simulink model "untitl3ed"  (R2021a)
settings: Solver=VariableStepAuto  StartTime=0.0  StopTime=10  RelTol=1e-3
undefined symbols (not defined in the file or in its folder): DiscIntNeverNeededParam, Ion, Lithium, sigbuilder_block
libraries: spsCurrentMeasurementLib x3, spsControlledCurrentSourceLib x2, spspowerguiLib x1, spsBatteryLib x1, spsControlledVoltageSourceLib x1, spsDiodeLib x1, spsFuelCellStackLib x1, spsSeriesRLCBranchLib x1, pid_lib x1
settings Model: Creator=leonardopalacios  LastModifiedBy=leonardopalacios
settings SolverCC: ZeroCrossAlgorithm=Adaptive
settings DebuggingCC: IgnoredZcDiagnostic=none

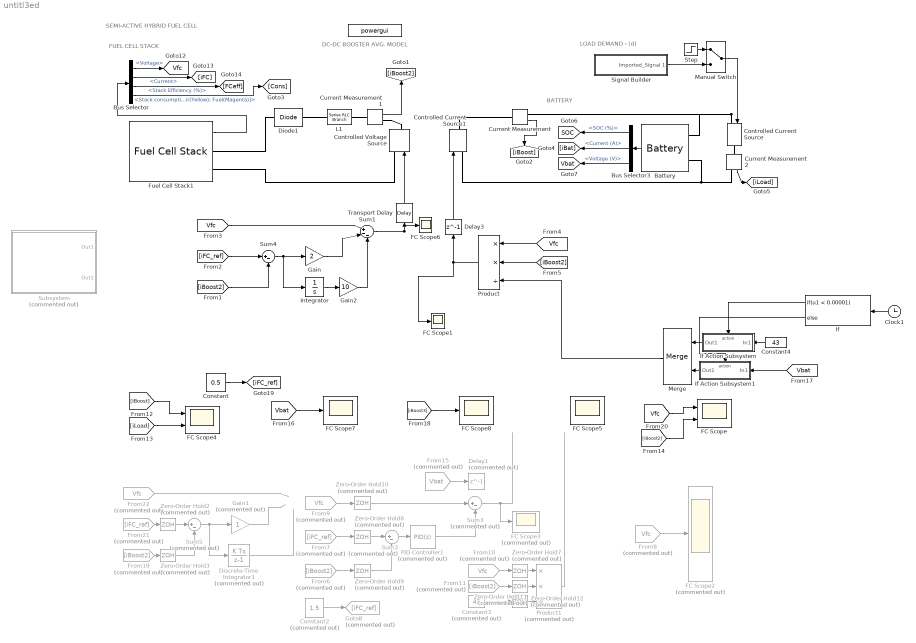
== system untitl3ed ==
  note: FUEL CELL STACK
  note: DC-DC BOOSTER AVG. MODEL
  note: BATTERY
  note: SEMI-ACTIVE HYBRID FUEL CELL
  note: LOAD DEMAND - (d)
  " " : spspowerguiLib/powergui  Priority=1  SimulationMode=Continuous  SampleTime=50e-6  frequency=60  Iterations=50  frequencyindice=0  Pbase=100e6  ErrMax=1e-4  UnitsV=kV  UnitsW=MW  buscounter=0  FunctionMessages=off  echomessages=off  EnableUseOfTLC=off  CurrentSourceSwitches=off  DisableSnubberDevices=off  DisableRonSwitches=off  DisableVfSwitches=off  DisplayEquations=off  AutomaticDiscreteSolvers=off  SolverType=Tustin/Backward Euler (TBE)  Interpol=off  ExternalGateDelay=off  methode=off  Ts=10  x0status=blocks  SPID=off  SwTol=0  HookPort=off  NonlinearTolerance=1e-4  nMaxIteration=100  ContinueOnMaxIteration=off  RestoreLinks=warning  ResistiveCurrentMeasurement=off  Frange=[0:2:500]  Ylog=off  Xlog=on  ShowGrid=off  save=off  variable=ZData  structure=0  ZoomFFT=off  StartTime=0.0  cycles=1  DisplayStyle=1  fundamental=60  FreqAxis=off  MaxFrequency=1000  frequencyindicesteady=1  RmsSteady=1  display=off
  Battery : spsBatteryLib/Battery  BatType=Lithium-Ion  ShowTempParam=off  ThermalPreset=no  ShowAgeParam=off  NomV=40  NomQ=2.2  SOC=50  Batt_Tr=30  PresetModel=on  MaxQ=2.2  MinV=30  FullV=46.5595  Dis_rate=0.95652  R=0.18182  Normal_OP=1.9896  expZone="[43.2154     0.108087]"  current=[6.5 13 32.5]  Units=Time  Tci=20  NomT=25  T2=0  MaxQ2=2.208  FullV2=3.45  Normal_OP2=2.8  expZone2="[3.22        0.23]"  Rca=0.6  ti=1000  Dp=0  Neq0=0  Tsim=1e6  Ta1=25  Qeol=5.4*0.9  Reol=0.013333*1.2  Char_age=[2.3478, 3]  Dis_age=[2.3478, 10]  N1=1500  N2=10500  N3=1000  N4=1400  Ta2=45  N5=950
  Bus Selector : BusSelector  OutputSignals=Voltage,Current,Stack Efficiency (%),Stack consumption (Standard lpm) [Air(Yellow); Fuel(Magenta)]
  Bus Selector3 : BusSelector  OutputSignals=SOC (%),Current (A),Voltage (V)
  Clock1 : Clock
  Constant : Constant  Value=0.5
  Constant2 : Constant  Commented=on  Value=1.5
  Constant3 : Constant  Commented=on  Value=43
  Constant4 : Constant  Value=43
  Controlled Current Source : spsControlledCurrentSourceLib/Controlled Current Source  Initialize=off  Source_Type=DC  Amplitude=0  Phase=0  Frequency=0  Measurements=Current
  Controlled Current Source1 : spsControlledCurrentSourceLib/Controlled Current Source  Initialize=on  Source_Type=DC  Amplitude=0  Phase=0  Frequency=0  Measurements=Current
  Controlled Voltage Source : spsControlledVoltageSourceLib/Controlled Voltage Source  Initialize=on  Source_Type=DC  Amplitude=32.5  Phase=0  Frequency=0  Measurements=None
  Current Measurement : spsCurrentMeasurementLib/Current Measurement  PhasorSimulation=off  OutputType=Complex  PSBequivalent=0
  Current Measurement1 : spsCurrentMeasurementLib/Current Measurement  PhasorSimulation=off  OutputType=Complex  PSBequivalent=0
  Current Measurement2 : spsCurrentMeasurementLib/Current Measurement  PhasorSimulation=off  OutputType=Complex  PSBequivalent=0
  Delay1 : Delay  Commented=on  DelayLength=1
  Delay3 : Delay  DelayLength=1
  Diode1 : spsDiodeLib/Diode  Ron=0.001  Lon=0  Vf=0.8  IC=0  UseSnubber=off  Rs=500  Cs=250e-9  Measurements=off
  Discrete-Time Integrator1 : DiscreteIntegrator  Commented=on  gainval=3  SampleTime=-1  ICPrevOutput=DiscIntNeverNeededParam  ICPrevScaledInput=DiscIntNeverNeededParam
  FC Scope : Scope  NumInputPorts=2
  FC Scope{1,5..8} (5 alike) : Scope
  FC Scope2 : Scope  Commented=on
  FC Scope3 : Scope  Commented=on
  FC Scope4 : Scope  NumInputPorts=2
  From{8..10,22} (4 alike) : From  Commented=on  GotoTag=Vfc  TagVisibility=global
  From11 : From  Commented=on  GotoTag=iBoost2
  From15 : From  Commented=on  GotoTag=Vbat  TagVisibility=global
  From19 : From  Commented=on  GotoTag=iBoost2
  From21 : From  Commented=on  GotoTag=iFC_ref
  From6 : From  Commented=on  GotoTag=iBoost2
  From7 : From  Commented=on  GotoTag=iFC_ref
  Fuel Cell Stack1 : spsFuelCellStackLib/Fuel Cell Stack  PresetModel=No (User-Defined)  FcType=0  Detailed=Detailed  Eoc="[18  15]"  NomVI="[4        12.5]"  EndVI="[5   12]"  Nc=20  n=46  TOp=25  AirFr=20  SuppPress="[0.35           0.3]"  Comp="[99.95           21            1]"  SignX=off  SignY=off  FlowRateH2=off  FlowRateAir=off  SystemTemp=off  SystemPH2=off  SystemPAir=off  FCDyn=off  FC_tau=1  Peak_O2=80  V_Under=10
      settings: SourceProductBaseCode=PS
  Gain : Gain  Gain=2
  Gain1 : Gain  Commented=on
  Gain2 : Gain  Gain=10
  Goto8 : Goto  Commented=on  GotoTag=iFC_ref
  If : If  IfExpression=u1 < 0.00001
  If Action Subsystem : Subsystem  TreatAsAtomicUnit=on
  If Action Subsystem1 : Subsystem  TreatAsAtomicUnit=on
  Integrator : Integrator
  L1 : spsSeriesRLCBranchLib/Series RLC Branch  LConnTagsString=__new0  RConnTagsString=__new0  BranchType=L  Resistance=1e5  Inductance=100e-3  SetiL0=off  InitialCurrent=0  Capacitance=1e-6  Setx0=off  InitialVoltage=0  Measurements=None
  Manual Switch : ManualSwitch
  Merge : Merge
  PID Controller1 : pid_lib/PID Controller  Commented=on  Controller=PID  Form=Parallel  TimeDomain=Discrete-time  UseExternalTs=off  SampleTime=-1  IntegratorMethod=Forward Euler  FilterMethod=Forward Euler  ControllerParametersSource=internal  P=1  I=10  D=0  UseFilter=on  N=100  TunerSelectOption=Transfer Function Based (PID Tuner App)  InitialConditionSource=internal  InitialConditionForIntegrator=0  InitialConditionForFilter=0  DifferentiatorICPrevScaledInput=0  ExternalReset=none  TrackingMode=off  Kt=1  LimitOutput=off  SatLimitsSource=internal  UpperSaturationLimit=inf  LowerSaturationLimit=-inf  LinearizeAsGain=on  AntiWindupMode=none  Kb=1  POutMin=[]  POutMax=[]  IOutMin=[]  IOutMax=[]  DOutMin=[]  DOutMax=[]  NOutMin=[]  NOutMax=[]  SumOutMin=[]  SumOutMax=[]  SaturationOutMin=[]  SaturationOutMax=[]  PParamMin=[]  PParamMax=[]  IParamMin=[]  IParamMax=[]  DParamMin=[]  DParamMax=[]  NParamMin=[]  NParamMax=[]  KbParamMin=[]  KbParamMax=[]  KtParamMin=[]  KtParamMax=[]  KbOutMin=[]  KbOutMax=[]  KtOutMin=[]  KtOutMax=[]  IntegratorOutMin=[]  IntegratorOutMax=[]  FilterOutMin=[]  FilterOutMax=[]  SumI1OutMin=[]  SumI1OutMax=[]  SumI2OutMin=[]  SumI2OutMax=[]  SumI3OutMin=[]  SumI3OutMax=[]  SumI4OutMin=[]  SumI4OutMax=[]  SumDOutMin=[]  SumDOutMax=[]  DifferentiatorOutMin=[]  DifferentiatorOutMax=[]  FilterDiffOutCoefMin=[]  FilterDiffOutCoefMax=[]  ReciprocalOutMin=[]  ReciprocalOutMax=[]  SumDenOutMin=[]  SumDenOutMax=[]  SumNumOutMin=[]  SumNumOutMax=[]  DivideOutMin=[]  DivideOutMax=[]  UdiffTsProdOutMin=[]  UdiffTsProdOutMax=[]  NTsProdOutMin=[]  NTsProdOutMax=[]  UintegralTsProdOutMin=[]  UintegralTsProdOutMax=[]  UngainTsProdOutMin=[]  UngainTsProdOutMax=[]  IntegratorContinuousStateAttributes=''  IntegratorStateMustResolveToSignalObject=off  IntegratorRTWStateStorageClass=Auto  FilterContinuousStateAttributes=''  FilterStateMustResolveToSignalObject=off  FilterRTWStateStorageClass=Auto  ParallelPVariant=InternalParameters  IdealPVariant=Disabled  IVariant=InternalParameters  DVariant=InternalParameters  IntegratorVariant=Discrete  SatVariant=Disabled  AWVariant=Passthrough  PCopyVariant=Disabled  TRVariant=Disabled  FdbkBlocksVariant=Forward  IdealPFdbkVariant=Disabled  SatFdbkVariant=Disabled  DerivativeFilterVariant=ForwardEulerFilter  NVariant=InternalParameters  NCopyVariant=Disabled  FilterICVariant=InternalICsFilter  IntegratorICVariant=InternalICs  ExternalResetVariant=Disabled  TRSumVariant=Passthrough  SumFdbkVariant=Disabled  SumVariant=Sum_PID  TsampFilterVariant=InternalTs  TsampNgainVariant=Passthrough  TsampIntegralVariant=Passthrough  ExternalSaturationOutDataTypeStr=Inherit: Same as second input
  Product : Product  Inputs=**/
  Product1 : Product  Commented=on  Inputs=**/
  Signal Builder : Subsystem  Tag=STV Subsys  LoadFcn=sigbuilder_block('load');  StartFcn=sigbuilder_block('start');  StopFcn=sigbuilder_block('stop');  ClipboardFcn=sigbuilder_block('clipboard');  mask(Sigbuilder block){tuvar=[0:10]}
      mask help: Simulink:masks:SigbuilderBlock_MD
      mask init:
      | if ~strcmp(get_param(bdroot(gcbh),'SimulationStatus'),'stopped') tuvar = sigbuilder_block('maskInit'); end
      settings: CopyFcn=sigbuilder_block('copy');  DeleteFcn=sigbuilder_block('delete');  ModelCloseFcn=sigbuilder_block('modelClose');  PreSaveFcn=sigbuilder_block('preSave');  PauseFcn=sigbuilder_block('pause');  ContinueFcn=sigbuilder_block('continue');  NameChangeFcn=sigbuilder_block('namechange');  OpenFcn=sigbuilder_block('open',[214 20 1706 550 ]);  CloseFcn=sigbuilder_block('close');
      mask Display: plot(0, 0, 100, 100,[2, 2, 32, 32, 2], [68, 8, 8, 68, 68],[32, 2], [38, 38], [32, 19, 2],[53, 60, 44], [32, 17, 17, 2],[16, 16, 31, 31]);txt = getActiveGroup(gcbh);text(2, 100, txt,'verticalAlignment', 'top');
  Step : Step  Time=0  After=0.6  SampleTime=0
  Subsystem : Subsystem  Commented=on
  Sum1 : Sum  Inputs=|+--
  Sum2 : Sum  Commented=on  Inputs=|+-
  Sum3 : Sum  Commented=on  Inputs=|+-
  Sum4 : Sum  Inputs=|+-
  Sum5 : Sum  Commented=on  Inputs=|+-
  Transport Delay : TransportDelay  DelayTime=0.00001
  Zero-Order Hold{2..3,7..12} (8 alike) : ZeroOrderHold  Commented=on  SampleTime=-1
  tag scope: SOC=global, Vbat=global, Vfc=global
  wires:
  Bus Selector3/1 -> [SOC]  "<SOC (%)>"
  Step/1 -> Manual Switch/1
  Current Measurement/1 -> [iBoost]
  Current Measurement2/1 -> [iLoad]
  Bus Selector/1 -> [Vfc]  "<Voltage>"
  Bus Selector/3 -> [FCeff]  "<Stack Efficiency (%)>"
  Signal Builder/1(Imported_Signal 1) -> Manual Switch/2
  Fuel Cell Stack1/1 -> Bus Selector/1
  Battery/1 -> Bus Selector3/1
  Manual Switch/1 -> Controlled Current Source/1
  Bus Selector3/2 -> [iBat]  "<Current (A)>"
  Bus Selector3/3 -> [Vbat]  "<Voltage (V)>"
  Bus Selector/4 -> [Cons]  "<Stack consumption (Standard lpm) [Air(Yellow); Fuel(Magenta)]>"
  Bus Selector/2 -> [iFC]  "<Current>"
  [Vfc] -> Sum1/1
  Constant/1 -> [iFC_ref]
  Product/1 -> Delay3/1, FC Scope1/1
  [Vfc] -> FC Scope/1
  From8/1 -> FC Scope2/1
  From10/1 -> Zero-Order Hold7/1
  Zero-Order Hold8/1 -> Sum2/1
  Zero-Order Hold9/1 -> Sum2/2
  Sum3/1 -> FC Scope3/1
  Zero-Order Hold11/1 -> Product1/2
  From6/1 -> Zero-Order Hold9/1
  From7/1 -> Zero-Order Hold8/1
  Zero-Order Hold12/1 -> Product1/3
  From9/1 -> Zero-Order Hold10/1
  Constant3/1 -> Zero-Order Hold12/1
  Sum2/1 -> PID Controller1/1
  PID Controller1/1 -> Sum3/2
  Product1/1 -> ?
  Zero-Order Hold10/1 -> Sum3/1
  Constant2/1 -> Goto8/1
  From11/1 -> Zero-Order Hold11/1
  Zero-Order Hold7/1 -> Product1/1
  Sum4/1 -> Integrator/1, Gain/1
  [iFC_ref] -> Sum4/1
  [iBoost2] -> Sum4/2
  [iBoost] -> FC Scope4/1
  [iLoad] -> FC Scope4/2
  [iBoost2] -> FC Scope/2
  From15/1 -> Delay1/1
  Integrator/1 -> Gain2/1
  [Vbat] -> FC Scope7/1
  Clock1/1 -> If/1
  Constant4/1 -> If Action Subsystem/1(In1)
  If/1 -> If Action Subsystem/Action
  If Action Subsystem/1(Out1) -> Merge/1
  If/2 -> If Action Subsystem1/Action
  If Action Subsystem1/1(Out1) -> Merge/2
  Merge/1 -> Product/3
  [Vbat] -> If Action Subsystem1/1(In1)
  Delay3/1 -> Controlled Current Source1/1
  [Vfc] -> Product/1
  [iBoost2] -> Product/2
  [iBoost3] -> FC Scope8/1
  From21/1 -> Zero-Order Hold2/1
  Zero-Order Hold3/1 -> Sum5/2
  From22/1 -> ?
  From19/1 -> Zero-Order Hold3/1
  Zero-Order Hold2/1 -> Sum5/1
  Gain1/1 -> ?
  Sum5/1 -> Discrete-Time Integrator1/1, Gain1/1
  Discrete-Time Integrator1/1 -> ?
  Sum1/1 -> FC Scope6/1, Transport Delay/1
  Current Measurement1/1 -> [iBoost2]
  Gain2/1 -> Sum1/3
  Gain/1 -> Sum1/2
  Transport Delay/1 -> Controlled Voltage Source/1
  connections:
  Controlled Current Source/LConn1 -- Current Measurement/RConn1 -- Battery/LConn1
  Battery/LConn2 -- Controlled Current Source1/LConn1 -- Current Measurement2/RConn1
  Controlled Current Source/RConn1 -- Current Measurement2/LConn1
  Fuel Cell Stack1/RConn1 -- Diode1/LConn1
  L1/LConn1 -- Diode1/RConn1
  Controlled Current Source1/RConn1 -- Current Measurement/LConn1
  Current Measurement1/LConn1 -- L1/RConn1
  Current Measurement1/RConn1 -- Controlled Voltage Source/RConn1
  Controlled Voltage Source/LConn1 -- Fuel Cell Stack1/RConn2

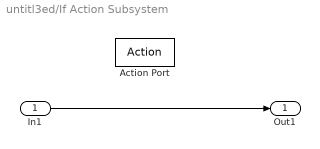
== system untitl3ed/If Action Subsystem ==
  In1 : Inport
  Action Port : ActionPort  ActionPortLabel=if(u1 < 0.00001)
  Out1 : Outport
  wires:
  In1/1 -> Out1/1

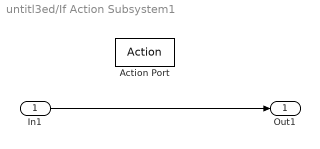
== system untitl3ed/If Action Subsystem1 ==
  In1 : Inport
  Action Port : ActionPort  ActionPortLabel=else
  Out1 : Outport
  wires:
  In1/1 -> Out1/1

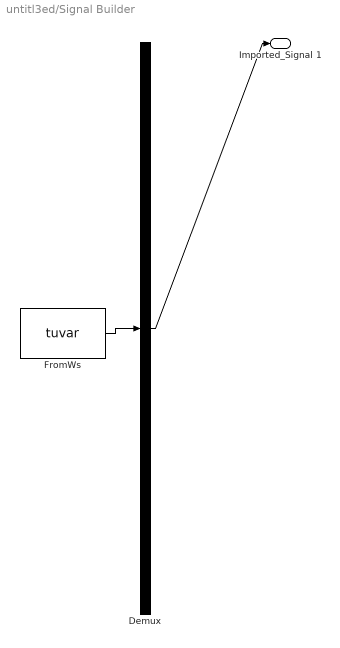
== system untitl3ed/Signal Builder ==
  Demux : Demux  Tag=STV Demux  Outputs=1
      settings: DisplayOption=none
  FromWs : FromWorkspace  Tag=STV FromWs  VariableName=tuvar
      SigBuilderData=|
      | common.afterFinalStr = 'Extrapolate'
      | common.sampleTime = 0
      | dataSet.timeRange = [0 1498.3]
      | dataSet.name = 'Combi12'
      | sbobj.Name = 'Signal Builder'
      | sbobj.Groups.Name = 'Combi12'
      | sbobj.Groups.Signals.Name = 'Imported_Signal 1'
      | sbobj.Groups.Signals.XData = [0 0.1 0.2 0.3 0.4 0.5 0.6 0.7 0.8 0.9 1 1.1 ... (14984 elements, 1x14984)]
      | sbobj.Groups.Signals.YData = [1.0569 1.1309 1.171 1.162 0.9589 1.143 1.056 1.261 1.1779 1.1458 1.2318 1.238 ... (14984 elements, 1x14984)]
      | sbobj.Groups.TimeRange = [0 1498.3]
  Imported_Signal 1 : Outport  Tag=STV Outport
  wires:
  FromWs/1 -> Demux/1
  Demux/1 -> Imported_Signal 1/1

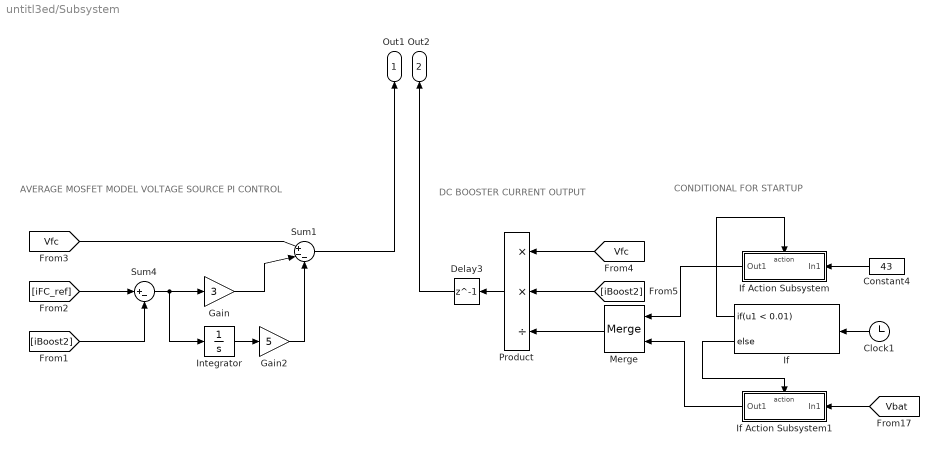
== system untitl3ed/Subsystem ==
  note: AVERAGE MOSFET MODEL VOLTAGE SOURCE PI CONTROL
  note: DC BOOSTER CURRENT OUTPUT
  note: CONDITIONAL FOR STARTUP
  Clock1 : Clock
  Constant4 : Constant  Value=43
  Delay3 : Delay  DelayLength=1
  Gain : Gain  Gain=3
  Gain2 : Gain  Gain=5
  If : If  IfExpression=u1 < 0.01
  If Action Subsystem : Subsystem  TreatAsAtomicUnit=on
  If Action Subsystem1 : Subsystem  TreatAsAtomicUnit=on
  Integrator : Integrator
  Merge : Merge
  Product : Product  Inputs=**/
  Sum1 : Sum  Inputs=|+--
  Sum4 : Sum  Inputs=|+-
  Out1 : Outport
  Out2 : Outport  Port=2
  wires:
  [Vbat] -> If Action Subsystem1/1(In1)
  Product/1 -> Delay3/1
  [Vfc] -> Sum1/1
  Gain/1 -> Sum1/2
  If/1 -> If Action Subsystem/Action
  [iBoost2] -> Sum4/2
  If/2 -> If Action Subsystem1/Action
  Sum4/1 -> Integrator/1, Gain/1
  Merge/1 -> Product/3
  Constant4/1 -> If Action Subsystem/1(In1)
  Integrator/1 -> Gain2/1
  Clock1/1 -> If/1
  Gain2/1 -> Sum1/3
  [iFC_ref] -> Sum4/1
  If Action Subsystem/1(Out1) -> Merge/1
  If Action Subsystem1/1(Out1) -> Merge/2
  Delay3/1 -> Out2/1
  [iBoost2] -> Product/2
  [Vfc] -> Product/1
  Sum1/1 -> Out1/1

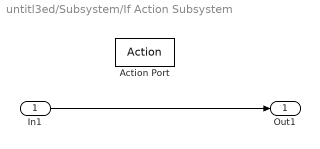
== system untitl3ed/Subsystem/If Action Subsystem ==
  In1 : Inport
  Action Port : ActionPort  ActionPortLabel=if(u1 < 0.01)
  Out1 : Outport
  wires:
  In1/1 -> Out1/1

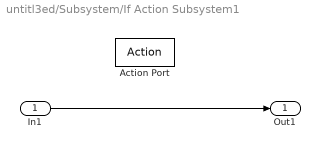
== system untitl3ed/Subsystem/If Action Subsystem1 ==
  In1 : Inport
  Action Port : ActionPort  ActionPortLabel=else
  Out1 : Outport
  wires:
  In1/1 -> Out1/1
